simulink model "FSM_parking_gate_broken"  (R2024a)
settings: Solver=FixedStepAuto  StartTime=0.0  StopTime=100  FixedStep=0.2  RelTol=1e-3
settings Model: PacingRate=2  Creator=ArriGE66  LastModifiedBy=Bocchio
settings ModelReferenceCC: EnableRefExpFcnMdlSchedulingChecks=on
settings RTWCC: GenCodeOnly=on  GPUComputeCapability=3.5

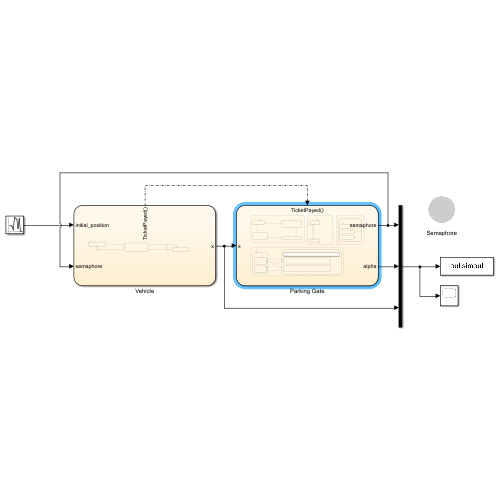
[thumbnail: Simulink's stored preview of the top-level diagram]
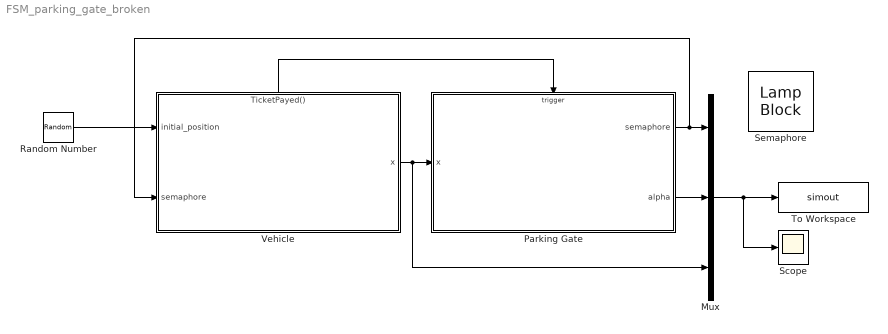
== system FSM_parking_gate_broken ==
  Mux : Mux  Inputs=3
  Parking Gate : Stateflow chart  TreatAsAtomicUnit=on
  Random Number : RandomNumber  Mean=-15  Variance=5  SampleTime=0.2
  Scope : Scope
  Semaphore : LampBlock  LabelPosition=Hide  Icon=Circle
  To Workspace : ToWorkspace  VariableName=simout  SampleTime=-1
  Vehicle : Stateflow chart  TreatAsAtomicUnit=on
      settings: PortSchema="{\"entries\":[{\"content\":{\"sides\":[{\"content\":{\"connectorIds\":[\"In1\",\"In2\"]},\"type\":\"ConnectorPlacement.EquallySpacedRectSide\",\"uuid\":\"85a5b07b-c6f7-4947-b221-d7458c14565e\"},{\"content\":{\"connectorIds\":[\"Out1\"],\"side\":\"RIGHT\"},\"type\":\"ConnectorPlacement.EquallySpacedRectSide\",\"uuid\":\"3e041a51-0a4a-4033-b8dc-49f4e7e27dc6\"},{\"content\":{\"connectorIds\":[\"Out2\"],\"side\":\"TOP\"},\"type\":\"ConnectorPlacement.EquallySpacedRectSide\",\"uuid\":\"156f6d46-69d8-4fb2-87cf-617a69469b2b\"},{\"content\":{\"side\":\"BOTTOM\"},\"type\":\"ConnectorPlacement.EquallySpacedRectSide\",\"uuid\":\"56f1fba6-ba20-4939-8692-e6d2650d2182\"}]},\"type\":\"ConnectorPlacement.EquallySpacedConnector\",\"uuid\":\"08d1f58e-a06b-4760-ab76-801cec63d8c4\"}],\"packageUris\":[\"http://schema.mathworks.com/mf0/Connector/R2020b\"],\"version\":\"1.0\"}"
  wires:
  Random Number/1 -> Vehicle/1(initial_position)
  Mux/1 -> Scope/1, To Workspace/1
  Vehicle/2(TicketPayed()) -> Parking Gate/Trigger
  Vehicle/1(x) -> Parking Gate/1(x), Mux/3
  Parking Gate/1(semaphore) -> Vehicle/2(semaphore), Mux/1
  Parking Gate/2(alpha) -> Mux/2

== stateflow chart FSM_parking_gate_broken/Vehicle ==
  state Spawning
    entry: x = initial_position;
  state Driving
    during:
    v = min(abs(x), 30/3.6)  + 10e-2;
    x = min(x + v*dt, checkpoint);
  state Waiting
    entry: send(TicketPayed);
  (default) -> Spawning
  Driving -> Waiting [order 1] : [x == checkpoint]
  Spawning -> Driving : {checkpoint = gate_pos;}
  (junction 233) -> Spawning
  Waiting -> Driving : [semaphore == 3]
      | / {checkpoint = +inf;}
  Driving -> (junction 233) [order 2] : after(10, sec)
  data: initial_position input double; dt constant double =0.2; v local double; x output double; checkpoint local double; gate_pos constant double =0; semaphore input
  events: TicketPayed output FUNCTION_CALL_EVENT

== stateflow chart FSM_parking_gate_broken/Parking Gate ==
  settings: executeAtInitialization=1
  state Controller [parallel]
    settings: executionOrder=1
    state Idling
    state GateOpening
      entry:
      %send(Yellow, Semaphore)
      send(Raise, Gate)
    state GateClosing
      entry:
      send(Lower, Gate)
      send(Red, Semaphore)
    state WaitingClearance
      entry: send(Green, Semaphore)
    (default) -> Controller.Idling
    Controller.Idling -> GateOpening : TicketPayed
    GateClosing -> Controller.Idling : [in(Gate.Idling.GateDown)]
    GateOpening -> WaitingClearance : [in(Gate.Idling.GateUp)]
    WaitingClearance -> GateClosing : [in(PhotoCell.Free)]
  state PhotoCell [parallel]
    settings: executionOrder=3
    state Free
    state Occupied
    (default) -> Free
    Occupied -> Free : [
        |   x<=(gate_x - 50e-2) || ...
        |   x>=(gate_x + car_length)
        | ]
    Free -> Occupied : [
        |   x>(gate_x - 50e-2) && ...
        |   x<(gate_x + car_length)
        | ]
  state Semaphore [parallel]
    settings: executionOrder=2
    state On
      state Red
        entry: semaphore = 1;
      state Yellow
        entry: semaphore = 2;
      state Green
        entry: semaphore = 3;
      (default) -> Red
      On -> Red [order 1] : Red
      On -> Yellow [order 2] : Yellow
      On -> Green [order 3] : Green
  state Gate [parallel]
    settings: executionOrder=4
    state Moving
      state Raising
        entry: [time, alphas] = computeTrapezoidalProfile(alpha, 90, max_omega, max_omega_dot);
        during: alpha = interp1(time, alphas, elapsed(sec), 'nearest', 'extrap');
      state Lowering
        entry: [time, alphas] = computeTrapezoidalProfile(alpha, 0, max_omega, max_omega_dot);
        during: alpha = interp1(time, alphas, elapsed(sec), 'nearest', 'extrap');
    state Idling
      state GateDown
        entry: alpha = 0;
      state GateUp
        entry: alpha = 90;
      (default) -> GateDown
    (default) -> Gate.Idling
    GateDown -> Raising : Raise
    Raising -> GateUp : [alpha == 90]
    Lowering -> GateDown : [alpha == 0]
    GateUp -> Lowering : Lower
  data: pos_current function_input; pos_target function_input; max_vel function_input; max_acc function_input; t_vec function_output; x_vec function_output; semaphore output; max_omega_dot constant double =1; max_omega constant double =4; car_length constant double =3; gate_x constant double =0; time local double; alphas local; x input double; alpha output
  events: Raise local FUNCTION_CALL_EVENT; Lower local FUNCTION_CALL_EVENT; TicketPayed input FUNCTION_CALL_EVENT; Red local FUNCTION_CALL_EVENT; Yellow local FUNCTION_CALL_EVENT; Green local FUNCTION_CALL_EVENT
  function [t_vec, x_vec] = computeTrapezoidalProfile(pos_current, pos_target, max_vel, max_acc):
    | function [t_vec, x_vec] = computeTrapezoidalProfile(pos_current, pos_target, max_vel, max_acc)
    | % COMPUTE_TRAPEZOIDAL_PROFILE Generates time and angle points for a trapezoidal profile
    | % At first checks if a trapezoidal profile is feasible or is necessary to
    | % fallback to a triangular one.
    | 
    | delta_pos = pos_target - pos_current;
    | time_acc_phase = max_vel / max_acc;
    | delta_pos_acc_phase = 0.5 * max_acc * time_acc_phase^2;
    | 
    | if 2 * delta_pos_acc_phase < abs(delta_pos)
    |     % Trapezoidal profile
    |     t1 = time_acc_phase;
    |     t2 = (abs(delta_pos) - 2 * delta_pos_acc_phase) / max_vel;
    |     t3 = time_acc_phase;
    | else
    |     % Triangular profile
    |     max_vel = sqrt(abs(delta_pos) * max_acc);
    |     t1 = max_vel / max_acc;
    |     t2 = 0;
    |     t3 = max_vel / max_acc;
    | end
    | 
    | 
    | % Trapezoidal profile template (HP: s0 = 0, v0 = 0)
    | acc = max_acc * sign(delta_pos);
    | vel = max_vel * sign(delta_pos);
    | profile_template = @(t) ...
    |     (t <= t1) .*                             (1/2 * acc * t.^2) + ...
    |     (t > t1 & t <= (t1 + t2)) .*             (1/2 * acc * t1^2 + vel * (t - t1)) + ...
    |     (t > (t1 + t2) & t <= (t1 + t2 + t3)) .* (1/2 * acc * t1^2 + vel * t2 + vel * (t - (t2 + t1)) - 1/2 * acc * (t - (t1 + t2)).^2) + ...
    |     (t > (t1 + t2 + t3)) .*                  (1/2 * acc * t1^2 + vel * t2 + vel * t3 - 1/2 * acc * t3.^2);
    | 
    | % Profile generation
    | t_vec = linspace(0, t1 + t2 + t3, 100);
    | x_vec = profile_template(t_vec) + pos_current;
    | 
    | end
